simulink model "Con_N_Leader_SimNashDis_Joystick"  (Simulink 8.9)
settings: Solver=ode5  StartTime=0.0  StopTime=60  FixedStep=0.01  RelTol=1e-3  EnableMultiTasking=on
StartFcn:
  | %global sysd;
  | %global weight;
  | %[ ~,sysd ] = LG_lf_double_Leader(1/20);
  | %[ weight ] = LG_weight();
values from neighbouring files (symbols this model uses):
  Hu = -Hu    [LG_Nash_Sol_1st.m]
  Hv = -Hv    [LG_Nash_Sol_1st.m]
  Tx2 = eye(26)    [Main_Joystick.m]
libraries: aerolibanimutils x2
settings Model: Creator=GeoLee  LastModifiedBy=gmh_n
settings DataIOCC: LimitDataPoints=off  SignalLoggingSaveFormat=Dataset  SaveOutput=off  SaveTime=off
settings DebuggingCC: UnderspecifiedInitializationDetection=Simplified  MergeDetectMultiDrivingBlocksExec=error  FcnCallInpInsideContextMsg=error  StateNameClashWarn=none  InitInArrayFormatMsg=none
settings GRTTargetCC: CombineOutputUpdateFcns=on  GRTInterface=off

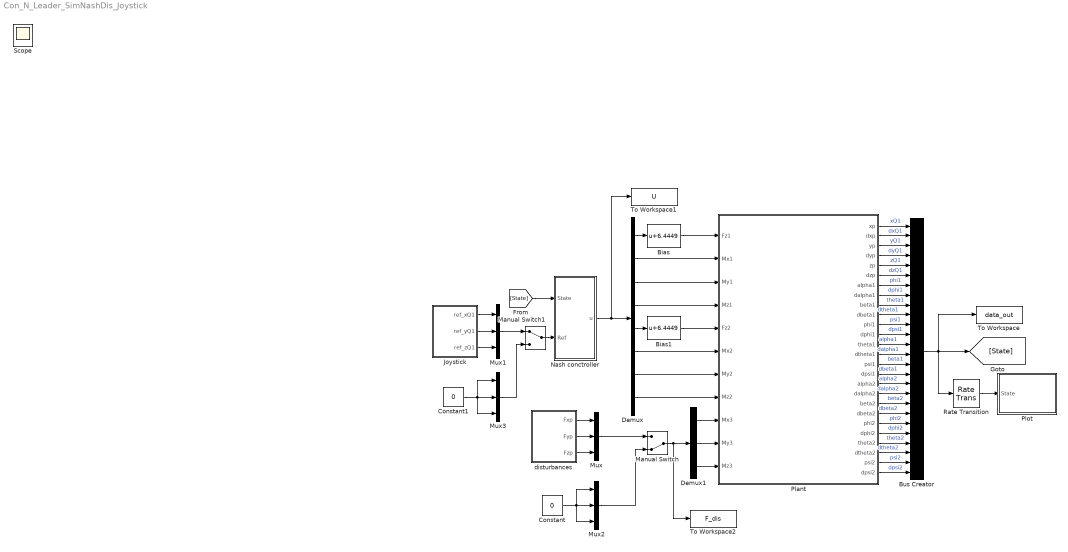
== system Con_N_Leader_SimNashDis_Joystick ==
  Bias : Bias  Bias=6.4449
  Bias1 : Bias  Bias=6.4449
  Bus Creator : BusCreator  Inputs=26
  Constant : Constant  Value=0
  Constant1 : Constant  Value=0
  Demux : Demux  Outputs=8
  Demux1 : Demux  Outputs=3
  Joystick : Subsystem
  Manual Switch : ManualSwitch  CurrentSetting=0
  Manual Switch1 : ManualSwitch
  Mux{,1..3} (4 alike) : Mux  Inputs=3
  Nash conctroller : Subsystem
  Plant : Subsystem  mask{xQ10=0, yQ10=0, zQ10=0, a10=0, b10=45, a20=180, b20=45}
      mask prompts: xQ10 "initial position of load xQ1"; yQ10 "initial position of load yQ1"; zQ10 "initial position of load zQ1"; a10 "alpha10(deg) (default: 0) (0~360)"; b10 "beta10(deg) (default: 45) (cannot be 0)"; a20 "alpha20(deg) (default: 180) (0~360)"; b20 "beta10(deg) (default: 45) (cannot be 0)"
      mask Display:
      | image('quads_double.png')
      | port_label('input', 1, 'Fz1')
      | port_label('input', 2, 'Mx1')
      | port_label('input', 3, 'My1')
      | port_label('input', 4, 'Mz1')
      | port_label('input', 5, 'Fz2')
      | port_label('input', 6, 'Mx2')
      | port_label('input', 7, 'My2')
      | port_label('input', 8, 'Mz2')
      | port_label('input', 9, 'Fxp')
      | port_label('input', 10, 'Fyp')
      | port_label('input', 11, 'Fzp')
      | 
      | port_label('output', 1, 'xQ1')
      | port_label('output', 2, 'dxQ1')
      | port_label('output', 3, 'yQ1')
      | port_label('output', 4, 'dyQ1')
      | port_label('output', 5, 'zQ1')
      | port_label('output', 6, 'dzQ1')
      | 
      | port_label('output', 7, 'phi1')
      | port_label('output', 8, 'dphi1')
      | port_label('output', 9, 'theta1')
      | port_label('output', 10, 'dtheta1')
      | port_label('output', 11, 'psi1')
      | port_label('output', 12, 'dpsi1')
      | 
      | port_label('output', 13, 'alpha1')
      | port_label('output', 14, 'dalpha1')
      | port_label('output', 15, 'beta1')
      | port_label('output', 16, 'dbeta1')
      | 
      | port_label('output', 17, 'alpha2')
      | port_label('output', 18, 'dalpha2')
      | port_label('output', 19, 'beta2')
      | port_label('output', 20, 'dbeta2')
      | port_label('output', 21, 'phi2')
      | port_label('output', 22, 'dphi2')
      | port_label('output', 23, 'theta2')
      | port_label('output', 24, 'dtheta2')
      | port_label('output', 25, 'psi2')
      | port_label('output', 26, 'dpsi2')
  Plot : Stateflow chart  TreatAsAtomicUnit=on
  Rate Transition : RateTransition  OutPortSampleTime=0.06
  To Workspace : ToWorkspace  VariableName=data_out  SampleTime=-1
  To Workspace1 : ToWorkspace  VariableName=U  SampleTime=-1
  To Workspace2 : ToWorkspace  VariableName=F_dis  SampleTime=-1
  disturbances : Subsystem
  Scope : Scope
  wires:
  Plant/1(xp) -> Bus Creator/1  "xQ1"
  Plant/2(dxp) -> Bus Creator/2  "dxQ1"
  Plant/3(yp) -> Bus Creator/3  "yQ1"
  Plant/4(dyp) -> Bus Creator/4  "dyQ1"
  Plant/5(zp) -> Bus Creator/5  "zQ1"
  Plant/6(dzp) -> Bus Creator/6  "dzQ1"
  Plant/7(alpha1) -> Bus Creator/7  "phi1"
  Plant/8(dalpha1) -> Bus Creator/8  "dphi1"
  Plant/9(beta1) -> Bus Creator/9  "theta1"
  Plant/10(dbeta1) -> Bus Creator/10  "dtheta1"
  Plant/11(phi1) -> Bus Creator/11  "psi1"
  Plant/12(dphi1) -> Bus Creator/12  "dpsi1"
  Plant/13(theta1) -> Bus Creator/13  "alpha1"
  Plant/14(dtheta1) -> Bus Creator/14  "dalpha1"
  Plant/15(psi1) -> Bus Creator/15  "beta1"
  Plant/16(dpsi1) -> Bus Creator/16  "dbeta1"
  Plant/17(alpha2) -> Bus Creator/17  "alpha2"
  Plant/18(dalpha2) -> Bus Creator/18  "dalpha2"
  Plant/19(beta2) -> Bus Creator/19  "beta2"
  Plant/20(dbeta2) -> Bus Creator/20  "dbeta2"
  Plant/21(phi2) -> Bus Creator/21  "phi2"
  Plant/22(dphi2) -> Bus Creator/22  "dphi2"
  Plant/23(theta2) -> Bus Creator/23  "theta2"
  Plant/24(dtheta2) -> Bus Creator/24  "dtheta2"
  Plant/25(psi2) -> Bus Creator/25  "psi2"
  Plant/26(dpsi2) -> Bus Creator/26  "dpsi2"
  Demux/2 -> Plant/2(Mx1)
  Demux/3 -> Plant/3(My1)
  Demux/4 -> Plant/4(Mz1)
  Demux/6 -> Plant/6(Mx2)
  Demux/8 -> Plant/8(Mz2)
  Demux/1 -> Bias/1
  Demux/5 -> Bias1/1
  Demux/7 -> Plant/7(My2)
  Bus Creator/1 -> Rate Transition/1, [State], To Workspace/1
  Manual Switch1/1 -> Nash conctroller/2(Ref)
  Joystick/3(ref_zQ1) -> Mux1/3
  [State] -> Nash conctroller/1(State)
  Joystick/1(ref_xQ1) -> Mux1/1
  Joystick/2(ref_yQ1) -> Mux1/2
  Rate Transition/1 -> Plot/1(State)
  Bias/1 -> Plant/1(Fz1)
  Bias1/1 -> Plant/5(Fz2)
  disturbances/1(Fxp) -> Mux/1
  disturbances/2(Fyp) -> Mux/2
  disturbances/3(Fzp) -> Mux/3
  Constant/1 -> Mux2/1, Mux2/2, Mux2/3
  Mux2/1 -> Manual Switch/2
  Mux/1 -> Manual Switch/1
  Demux1/1 -> Plant/9(Mx3)
  Demux1/2 -> Plant/10(My3)
  Demux1/3 -> Plant/11(Mz3)
  Manual Switch/1 -> To Workspace2/1, Demux1/1
  Mux3/1 -> Manual Switch1/2
  Constant1/1 -> Mux3/3, Mux3/2, Mux3/1
  Mux1/1 -> Manual Switch1/1
  Nash conctroller/1(u) -> To Workspace1/1, Demux/1

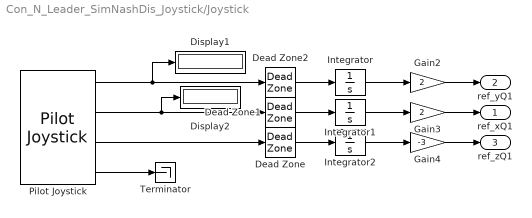
== system Con_N_Leader_SimNashDis_Joystick/Joystick ==
  Dead Zone : DeadZone  LowerValue=-0.1  UpperValue=0.1  SaturateOnIntegerOverflow=on
  Dead Zone1 : DeadZone  LowerValue=-0.1  UpperValue=0.1  SaturateOnIntegerOverflow=on
  Dead Zone2 : DeadZone  LowerValue=-0.1  UpperValue=0.1  SaturateOnIntegerOverflow=on
  Display1 : Display
  Display2 : Display
  Gain2 : Gain  Gain=2
  Gain3 : Gain  Gain=2
  Gain4 : Gain  Gain=-3
  Integrator : Integrator
  Integrator1 : Integrator
  Integrator2 : Integrator
  Pilot Joystick : aerolibanimutils/Pilot Joystick  JoystickID=Joystick1  OutputConfiguration=FourAxis  SampleTime=0.01
  Terminator : Terminator
  ref_xQ1 : Outport
  ref_yQ1 : Outport  Port=2
  ref_zQ1 : Outport  Port=3
  wires:
  Gain4/1 -> ref_zQ1/1
  Pilot Joystick/4 -> Terminator/1
  Gain3/1 -> ref_xQ1/1
  Pilot Joystick/2 -> Dead Zone1/1, Display2/1
  Gain2/1 -> ref_yQ1/1
  Integrator/1 -> Gain2/1
  Integrator1/1 -> Gain3/1
  Integrator2/1 -> Gain4/1
  Pilot Joystick/1 -> Dead Zone2/1, Display1/1
  Dead Zone1/1 -> Integrator1/1
  Dead Zone/1 -> Integrator2/1
  Dead Zone2/1 -> Integrator/1
  Pilot Joystick/3 -> Dead Zone/1

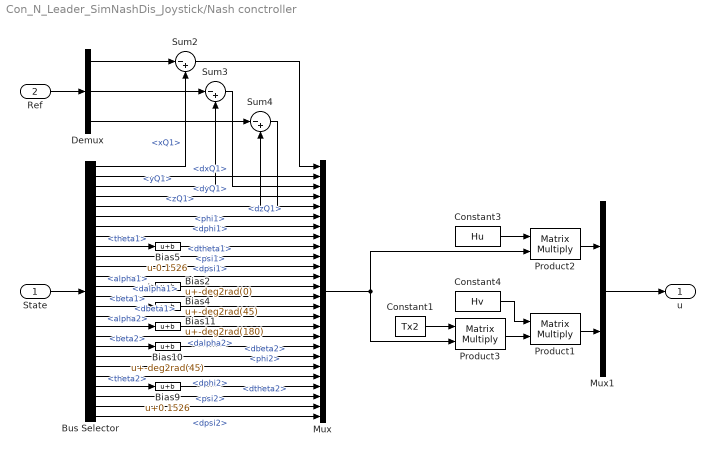
== system Con_N_Leader_SimNashDis_Joystick/Nash conctroller ==
  State : Inport
  Ref : Inport  Port=2
  Bias10 : Bias  Bias=-deg2rad(45)
  Bias11 : Bias  Bias=-deg2rad(180)
  Bias2 : Bias  Bias=-deg2rad(0)
  Bias4 : Bias  Bias=-deg2rad(45)
  Bias5 : Bias  Bias=-0.1526
  Bias9 : Bias  Bias=0.1526
  Bus Selector : BusSelector  OutputSignals=xQ1,dxQ1,yQ1,dyQ1,zQ1,dzQ1,phi1,dphi1,theta1,dtheta1,psi1,dpsi1,alpha1,dalpha1,beta1,dbeta1,alpha2,dalpha2,beta2,dbeta2,phi2,dphi2,theta2,dtheta2,psi2,dpsi2
  Constant1 : Constant  Value=Tx2
  Constant3 : Constant  Value=Hu
  Constant4 : Constant  Value=Hv
  Demux : Demux  Outputs=3
  Mux : Mux  Inputs=26
  Mux1 : Mux  Inputs=2
  Product1 : Product  Multiplication=Matrix(*)  RndMeth=Zero
  Product2 : Product  Multiplication=Matrix(*)  RndMeth=Zero
  Product3 : Product  Multiplication=Matrix(*)  RndMeth=Zero
  Sum2 : Sum  Inputs=|-+
  Sum3 : Sum  Inputs=|-+
  Sum4 : Sum  Inputs=|-+
  u : Outport
  wires:
  State/1 -> Bus Selector/1
  Bus Selector/1 -> Sum2/2  "<xQ1>"
  Bus Selector/2 -> Mux/2  "<dxQ1>"
  Bus Selector/3 -> Sum3/2  "<yQ1>"
  Bus Selector/4 -> Mux/4  "<dyQ1>"
  Bus Selector/5 -> Sum4/2  "<zQ1>"
  Bus Selector/6 -> Mux/6  "<dzQ1>"
  Bus Selector/7 -> Mux/7  "<phi1>"
  Bus Selector/8 -> Mux/8  "<dphi1>"
  Bus Selector/9 -> Bias5/1  "<theta1>"
  Bus Selector/10 -> Mux/10  "<dtheta1>"
  Bus Selector/11 -> Mux/11  "<psi1>"
  Bus Selector/12 -> Mux/12  "<dpsi1>"
  Bus Selector/13 -> Bias2/1  "<alpha1>"
  Bus Selector/14 -> Mux/14  "<dalpha1>"
  Bus Selector/15 -> Bias4/1  "<beta1>"
  Bus Selector/16 -> Mux/16  "<dbeta1>"
  Bus Selector/17 -> Bias11/1  "<alpha2>"
  Bus Selector/18 -> Mux/18  "<dalpha2>"
  Bus Selector/19 -> Bias10/1  "<beta2>"
  Bus Selector/20 -> Mux/20  "<dbeta2>"
  Bus Selector/21 -> Mux/21  "<phi2>"
  Bus Selector/22 -> Mux/22  "<dphi2>"
  Bus Selector/23 -> Bias9/1  "<theta2>"
  Bus Selector/24 -> Mux/24  "<dtheta2>"
  Bus Selector/25 -> Mux/25  "<psi2>"
  Bus Selector/26 -> Mux/26  "<dpsi2>"
  Bias5/1 -> Mux/9
  Bias9/1 -> Mux/23
  Bias4/1 -> Mux/15
  Bias10/1 -> Mux/19
  Bias2/1 -> Mux/13
  Bias11/1 -> Mux/17
  Sum2/1 -> Mux/1
  Demux/1 -> Sum2/1
  Demux/2 -> Sum3/1
  Demux/3 -> Sum4/1
  Sum3/1 -> Mux/3
  Sum4/1 -> Mux/5
  Ref/1 -> Demux/1
  Mux1/1 -> u/1
  Constant3/1 -> Product2/1
  Constant4/1 -> Product1/1
  Product1/1 -> Mux1/2
  Product2/1 -> Mux1/1
  Mux/1 -> Product2/2, Product3/2
  Product3/1 -> Product1/2
  Constant1/1 -> Product3/1

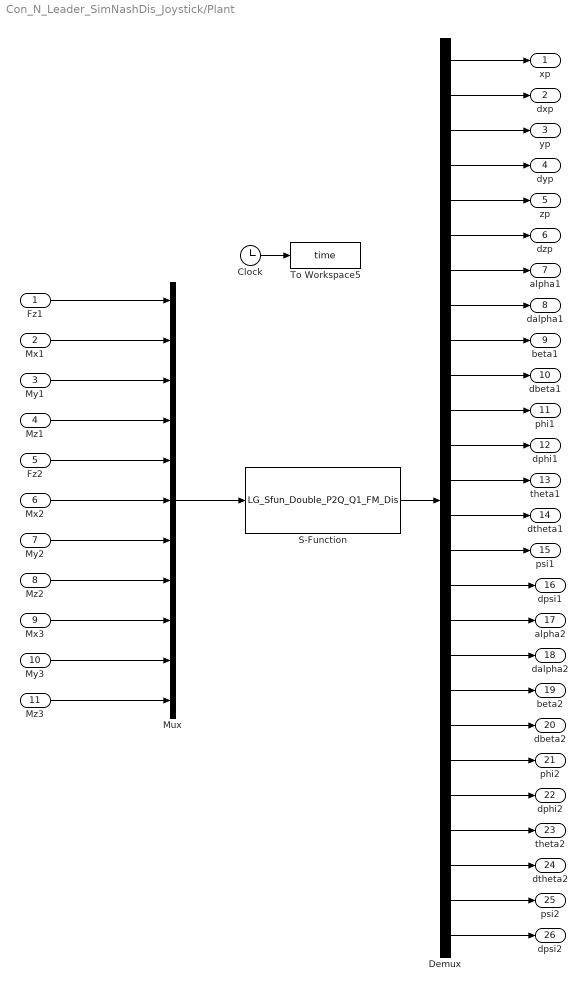
== system Con_N_Leader_SimNashDis_Joystick/Plant ==
  Fz1 : Inport
  Mx1 : Inport  Port=2
  My1 : Inport  Port=3
  Mz1 : Inport  Port=4
  Fz2 : Inport  Port=5
  Mx2 : Inport  Port=6
  My2 : Inport  Port=7
  Mz2 : Inport  Port=8
  Mx3 : Inport  Port=9
  My3 : Inport  Port=10
  Mz3 : Inport  Port=11
  Clock : Clock
  Demux : Demux  Outputs=26
  Mux : Mux  Inputs=11
  S-Function : S-Function  FunctionName=LG_Sfun_Double_P2Q_Q1_FM_Dis  Parameters=xQ10,yQ10,zQ10,a10,b10,a20,b20  SFunctionDeploymentMode=off  EnableBusSupport=off
  To Workspace5 : ToWorkspace  VariableName=time  SampleTime=-1
  xp : Outport
  dxp : Outport  Port=2
  yp : Outport  Port=3
  dyp : Outport  Port=4
  zp : Outport  Port=5
  dzp : Outport  Port=6
  alpha1 : Outport  Port=7
  dalpha1 : Outport  Port=8
  beta1 : Outport  Port=9
  dbeta1 : Outport  Port=10
  phi1 : Outport  Port=11
  dphi1 : Outport  Port=12
  theta1 : Outport  Port=13
  dtheta1 : Outport  Port=14
  psi1 : Outport  Port=15
  dpsi1 : Outport  Port=16
  alpha2 : Outport  Port=17
  dalpha2 : Outport  Port=18
  beta2 : Outport  Port=19
  dbeta2 : Outport  Port=20
  phi2 : Outport  Port=21
  dphi2 : Outport  Port=22
  theta2 : Outport  Port=23
  dtheta2 : Outport  Port=24
  psi2 : Outport  Port=25
  dpsi2 : Outport  Port=26
  wires:
  Demux/10 -> dbeta1/1
  My2/1 -> Mux/7
  Demux/24 -> dtheta2/1
  Demux/23 -> theta2/1
  Demux/22 -> dphi2/1
  Demux/21 -> phi2/1
  Demux/20 -> dbeta2/1
  Demux/19 -> beta2/1
  Demux/18 -> dalpha2/1
  Mz1/1 -> Mux/4
  Demux/16 -> dpsi1/1
  Demux/14 -> dtheta1/1
  Demux/15 -> psi1/1
  Mx2/1 -> Mux/6
  Demux/17 -> alpha2/1
  Demux/13 -> theta1/1
  Demux/12 -> dphi1/1
  Demux/8 -> dalpha1/1
  Demux/5 -> zp/1
  My1/1 -> Mux/3
  Demux/9 -> beta1/1
  Demux/6 -> dzp/1
  Demux/11 -> phi1/1
  Demux/25 -> psi2/1
  Demux/7 -> alpha1/1
  Demux/4 -> dyp/1
  Demux/3 -> yp/1
  Mx1/1 -> Mux/2
  Demux/1 -> xp/1
  Demux/2 -> dxp/1
  Demux/26 -> dpsi2/1
  Mz2/1 -> Mux/8
  S-Function/1 -> Demux/1
  Mux/1 -> S-Function/1
  Fz1/1 -> Mux/1
  Fz2/1 -> Mux/5
  Clock/1 -> To Workspace5/1
  Mx3/1 -> Mux/9
  My3/1 -> Mux/10
  Mz3/1 -> Mux/11

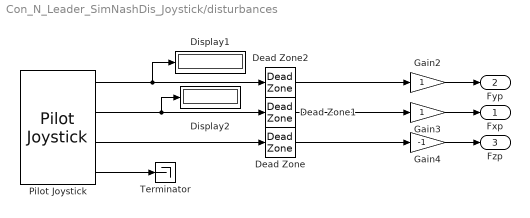
== system Con_N_Leader_SimNashDis_Joystick/disturbances ==
  Dead Zone : DeadZone  LowerValue=-0.1  UpperValue=0.1  SaturateOnIntegerOverflow=on
  Dead Zone1 : DeadZone  LowerValue=-0.1  UpperValue=0.1  SaturateOnIntegerOverflow=on
  Dead Zone2 : DeadZone  LowerValue=-0.1  UpperValue=0.1  SaturateOnIntegerOverflow=on
  Display1 : Display
  Display2 : Display
  Gain2 : Gain
  Gain3 : Gain
  Gain4 : Gain  Gain=-1
  Pilot Joystick : aerolibanimutils/Pilot Joystick  JoystickID=Joystick1  OutputConfiguration=FourAxis  SampleTime=0.01
  Terminator : Terminator
  Fxp : Outport
  Fyp : Outport  Port=2
  Fzp : Outport  Port=3
  wires:
  Pilot Joystick/3 -> Dead Zone/1
  Pilot Joystick/1 -> Display1/1, Dead Zone2/1
  Dead Zone/1 -> Gain4/1
  Dead Zone1/1 -> Gain3/1
  Dead Zone2/1 -> Gain2/1
  Gain2/1 -> Fyp/1
  Pilot Joystick/2 -> Display2/1, Dead Zone1/1
  Gain3/1 -> Fxp/1
  Pilot Joystick/4 -> Terminator/1
  Gain4/1 -> Fzp/1

== stateflow chart Plot ==
  state Plot
    entry:
    fig = ml.figure();
    phandles = ml.LG_plot_initial(fig,State);
    du:
    ml.LG_plot_update(fig,State,phandles);
  (default) -> Plot
  data: State input double size=26; fig local ml; phandles local ml
